simulink model "trainmodel"  (R2013a)
settings: Solver=ode4  StartTime=0.0  StopTime=100  FixedStep=1e-4  RelTol=1e-3
settings Model: Creator=ugurm  LastModifiedBy=ugurm

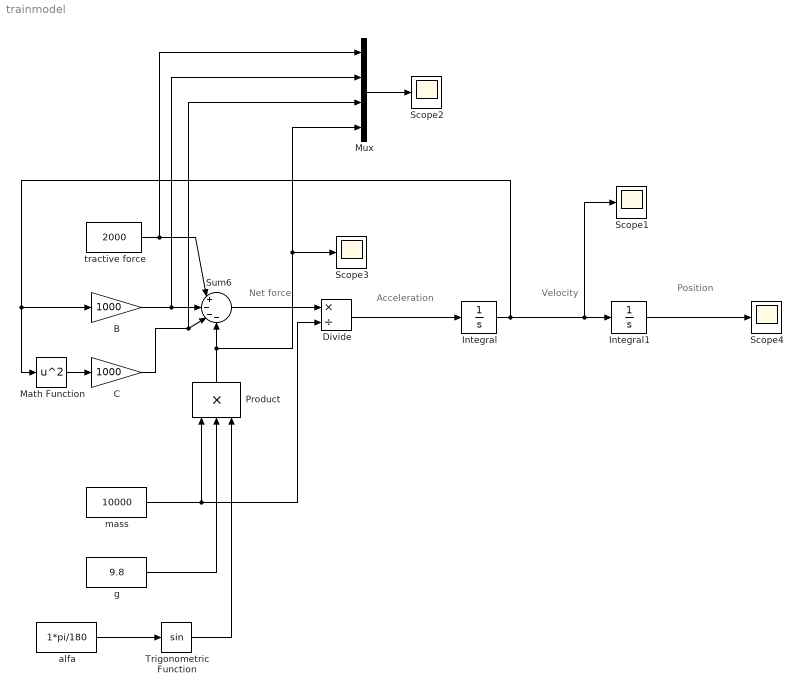
== system trainmodel ==
  note: Net force
  note: Acceleration
  note: Velocity
  note: Position
  B : Gain  Gain=1000
  C : Gain  Gain=1000
  Divide : Product  Inputs=*/
  Integral : TransferFcn  Denominator=[1 0]
  Integral1 : TransferFcn  Denominator=[1 0]
  Math Function : Math  Operator=square  SaturateOnIntegerOverflow=on
  Mux : Mux
  Product : Product  Inputs=3
  Scope{1..4} (4 alike) : Scope
      Scope1 settings: YMin=0  YMax=2.75
      Scope2 settings: YMin=0  YMax=200000
      Scope3 settings: YMin=0  YMax=20000  SaveName=ScopeData2
      Scope4 settings: YMin=0  YMax=1200  SaveName=ScopeData3
  Sum6 : Sum  Inputs=|+---
  Trigonometric Function : Trigonometry
  alfa : Constant  Value=1*pi/180
  g : Constant  Value=9.8
  mass : Constant  Value=10000
  tractive force : Constant  Value=2000
  wires:
  tractive force/1 -> Mux/1, Sum6/1
  B/1 -> Mux/2, Sum6/2
  C/1 -> Mux/3, Sum6/3
  Product/1 -> Scope3/1, Mux/4, Sum6/4
  mass/1 -> Divide/2, Product/1
  g/1 -> Product/2
  alfa/1 -> Trigonometric Function/1
  Trigonometric Function/1 -> Product/3
  Sum6/1 -> Divide/1
  Divide/1 -> Integral/1
  Integral/1 -> Scope1/1, Integral1/1, Math Function/1, B/1
  Math Function/1 -> C/1
  Integral1/1 -> Scope4/1
  Mux/1 -> Scope2/1
